simulink model "HW11_111205023_2017b"  (R2017b)
settings: Solver=VariableStepAuto  StartTime=0.0  StopTime=inf  RelTol=1e-3
libraries: commdigbbndpm3 x2, commfilt2 x2, commchan3 x1, commrandsrc3 x1, commutil2 x1, commrflib2 x1, dspsigops x1
settings Model: Creator=User  LastModifiedBy=User
settings DataIOCC: ReturnWorkspaceOutputs=on
settings DebuggingCC: UnconnectedInputMsg=none  UnconnectedOutputMsg=none  UnconnectedLineMsg=none  SFMachineParentedDataDiag=error
settings ModelReferenceCC: EnableRefExpFcnMdlSchedulingChecks=off
settings SFSimCC: SimUseLocalCustomCode=on
settings RTWCC: Description=Generic Real-Time Target  RTWUseLocalCustomCode=on

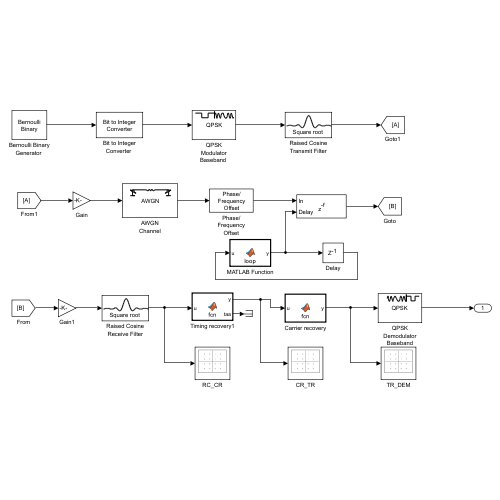
[thumbnail: Simulink's stored preview of the top-level diagram]
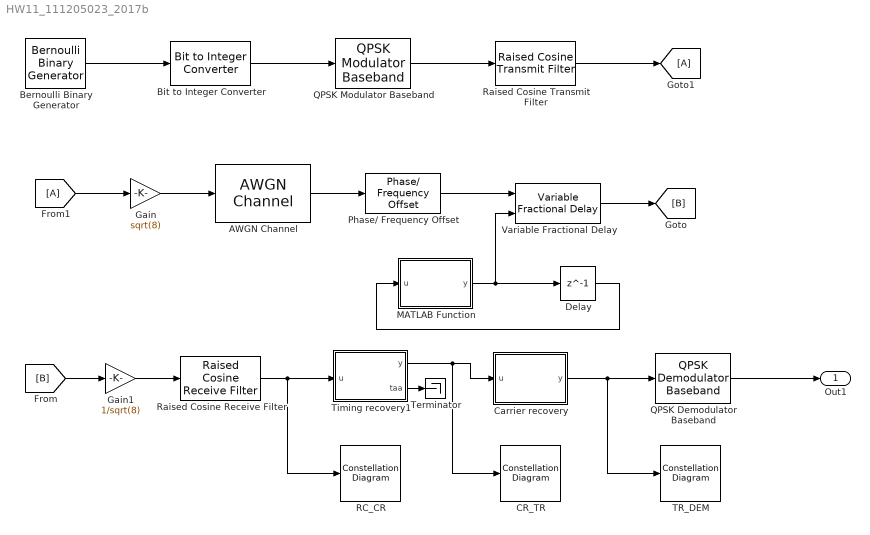
== system HW11_111205023_2017b ==
  AWGN Channel : commchan3/AWGN Channel  InputProcessing=Columns as channels (frame based)  seed=61  noiseMode="Signal to noise ratio  (Eb/No)"  EbNodB=20  EsNodB=10  SNRdB=10  bitsPerSym=1  Ps=1  Tsym=1  variance=1
  "Bernoulli Binary Generator " : commrandsrc3/Bernoulli Binary Generator  ProbabilityOfZero=0.5  SeedSource=Parameter  Seed=61  SampleTime=1  SamplesPerFrame=512  OutputDataType=double  SimulateUsing=Interpreted execution
  "Bit to Integer Converter " : commutil2/Bit to Integer Converter  nbits=2  bitOrder=MSB first  signedOutputValues=Unsigned  outDtype=Inherit via internal rule  outDtypeSigned=Inherit via internal rule
  CR_TR : ConstellationDiagram  DefaultConfigurationName=comm.scopes.ConstellationDiagramBlockCfg
  Carrier recovery : MATLAB Function  TreatAsAtomicUnit=on
  Delay : Delay  DelayLength=1  InitialCondition=0
  Gain : Gain  Gain=sqrt(8)
  Gain1 : Gain  Gain=1/sqrt(8)
  MATLAB Function : MATLAB Function  TreatAsAtomicUnit=on
  Phase/ Frequency Offset : commrflib2/Phase// Frequency Offset  phaseOffset=0  freqPort=off  freqOffset=4e-3
  QPSK Demodulator Baseband : commdigbbndpm3/QPSK Demodulator Baseband  OutType=Integer  DecType=Hard decision  VarSource=Dialog  Variance=1  Dec=Gray  Ph=pi/4  outDtype1=Inherit via internal rule  outDtype2=Inherit via internal rule  derotateFactorWordLen=16  derotateFactorDataTypeStr=Inherit: Same word length as input  derotateFactorLastDataTypeStr=Inherit: Same word length as input
  "QPSK Modulator Baseband " : commdigbbndpm3/QPSK Modulator Baseband  InType=Integer  Enc=Gray  Ph=pi/4  outDtype=double  outWordLen=16  outUDDataType=sfix(16)  outFracLenMode=Best precision  outFracLen=15  outDataTypeStr=double  outLastDataTypeStr=double
  RC_CR : ConstellationDiagram  DefaultConfigurationName=comm.scopes.ConstellationDiagramBlockCfg
  Raised Cosine Receive Filter : commfilt2/Raised Cosine Receive Filter  filtType=Square root  R=0.3  filtSpan=10  N=8  downFactor=1  downOffset=0  filterGain=1  InputProcessing=Columns as channels (frame based)  RateOptions=Allow multirate processing  framing=Mute  checkCoeff=off  variableName=rcRxFilt  currentFiltSpan=10  D=5  inputOffset=0  sampMode=Mute  saveAsFlag=0  rateMode=Downsampling  checkGain=Normalized  launchFVT=on  roundingMode=Floor  overflowMode=off  coeffDataTypeStr=Inherit: Same word length as input  coeffMin=[]  coeffMax=[]  coeffLastDataTypeStr=Inherit: Same word length as input  accumDataTypeStr=Inherit: Same as product output  accumLastDataTypeStr=Inherit: Same as product output  outputDataTypeStr=Inherit: Same as accumulator  outputMin=[]  outputMax=[]  outputLastDataTypeStr=Inherit: Same as accumulator
  Raised Cosine Transmit Filter : commfilt2/Raised Cosine Transmit Filter  filtType=Square root  R=0.3  filtSpan=10  N=8  filterGain=1  InputProcessing=Columns as channels (frame based)  RateOptions=Enforce single-rate processing  framing=Mute  checkCoeff=off  variableName=rcTxFilt  checkGain=Normalized  sampMode=Mute  saveAsFlag=0  currentFiltSpan=10  D=5  launchFVT=on  roundingMode=Floor  overflowMode=off  coeffDataTypeStr=Inherit: Same word length as input  coeffMin=[]  coeffMax=[]  coeffLastDataTypeStr=Inherit: Same word length as input  outputDataTypeStr=Inherit: Same as accumulator  outputMin=[]  outputMax=[]  outputLastDataTypeStr=Inherit: Same as accumulator
  TR_DEM : ConstellationDiagram  DefaultConfigurationName=comm.scopes.ConstellationDiagramBlockCfg
  Terminator : Terminator
  Timing recovery1 : MATLAB Function  TreatAsAtomicUnit=on
  Variable Fractional Delay : dspsigops/Variable Fractional Delay  mode=OBSOLETE  modeActive=Linear  L=4  FarrowL=4  R=10  alpha=1  dmax=100  InputProcessing=Columns as channels (frame based)  ic=0  noDFT=off  fallbackFIR=Clip to the minimum value necessary for centered kernel  fallbackFarrow=Clip to the minimum value necessary for centered kernel  roundingMode=Zero  overflowMode=off
  Out1 : Outport
  wires:
  "Bernoulli Binary Generator "/1 -> "Bit to Integer Converter "/1
  "Bit to Integer Converter "/1 -> "QPSK Modulator Baseband "/1
  "QPSK Modulator Baseband "/1 -> Raised Cosine Transmit Filter/1
  Gain/1 -> AWGN Channel/1
  Phase/ Frequency Offset/1 -> Variable Fractional Delay/1
  MATLAB Function/1(y) -> Variable Fractional Delay/2, Delay/1
  Delay/1 -> MATLAB Function/1(u)
  AWGN Channel/1 -> Phase/ Frequency Offset/1
  Variable Fractional Delay/1 -> [B]
  Raised Cosine Transmit Filter/1 -> [A]
  [A] -> Gain/1
  QPSK Demodulator Baseband/1 -> Out1/1
  Gain1/1 -> Raised Cosine Receive Filter/1
  [B] -> Gain1/1
  Timing recovery1/2(taa) -> Terminator/1
  Raised Cosine Receive Filter/1 -> RC_CR/1, Timing recovery1/1(u)
  Timing recovery1/1(y) -> CR_TR/1, Carrier recovery/1(u)
  Carrier recovery/1(y) -> TR_DEM/1, QPSK Demodulator Baseband/1

== matlab function HW11_111205023_2017b/Carrier recovery ==
  data: u input; y output size=260
function y = fcn(u)
    persistent er eri vco sk;
    if isempty(er)
         er = 0;
         eri = 0;
         vco = 0;
         sk = 0;
    end
    
    %% Initialize PLL
    n = length(u);
    alpha = 0.01;
    beta =  0.001;
    
    y = u;
    for a = 2:n
        % decision detect
        eri = u(a) * exp(-1i * vco);    

        % Detection (Decision boundary)
        if real(eri) >= 0
            bit_r = 1;
        else
            bit_r = -1;
        end
        if imag(eri) >= 0
            bit_i = 1;
        else
            bit_i = -1;
        end
  
        Ak = bit_r + i*bit_i;
    
        % phase detector
        er = angle((eri) * conj(Ak));
    
        % loop filter
        sk = (sk + (beta * er)) ;
        gk = alpha * er;
        ck = gk + sk;
        
        % VCO
        vco = vco + ck;
        y(a) = eri;
    end

    y(1) = u(1) * exp(-1i * vco);  
end

== matlab function HW11_111205023_2017b/MATLAB Function ==
  data: u input; y output
function y = loop(u)
    y = u+0.001;
end

== matlab function HW11_111205023_2017b/Timing recovery1 ==
  data: u input; y output size=260; taa output
function [y,taa] = fcn(u)
    persistent ta u_s;
    beta = 0.02;

    if isempty(ta)
        ta = 0;
        u_s = complex(zeros(4,1));
    end
    uu=[u_s;u];

    if (ta == 0)
        ta = 1;
    end
    y_a = uu(ta :8: end);
    y_m = uu(ta+4 :8: end);
    y_b = [uu(ta+8 :8: end);u(end)];

    e = beta*real((y_b(1:256) - y_a(1:256))'*y_m(1:256));
    y = y_m(1:256);
    ta = ta+sign(round(e));
    if (ta < 0)
        ta = ta+8;
    elseif (ta > 7)
        ta=ta-8;
    end

    u_s = uu(end-3:end);
    taa = ta;
end
